simulink subsystem "AGTF30"  (R2021b)
settings: Solver=VariableStepAuto  StartTime=0.0  StopTime=10.0  RelTol=1e-3
undefined symbols (not defined in the file): MWS
libraries: Lib_Solve_IterNRSolverJC_TMATS x1
settings Model: Creator=prbalm  LastModifiedBy=prbalm

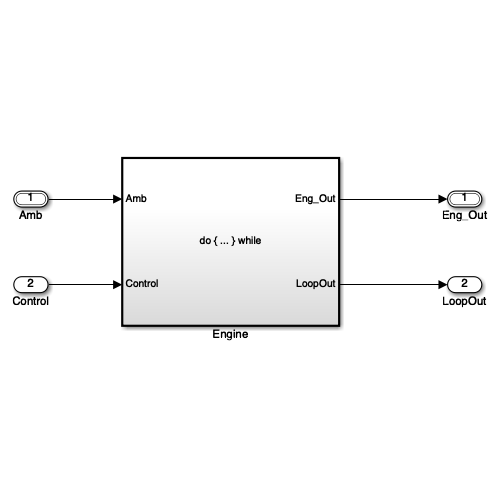
[thumbnail: Simulink's stored preview of the top-level diagram]
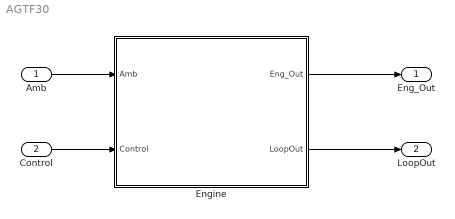
== system AGTF30 ==
  Amb : Inport
  Control : Inport  Port=2
  Engine : Subsystem
  Eng_Out : Outport  OutDataTypeStr=Bus: Eng_Bus
  LoopOut : Outport  Port=2
  wires:
  Engine/1(Eng_Out) -> Eng_Out/1
  Amb/1 -> Engine/1(Amb)
  Control/1 -> Engine/2(Control)
  Engine/2(LoopOut) -> LoopOut/1

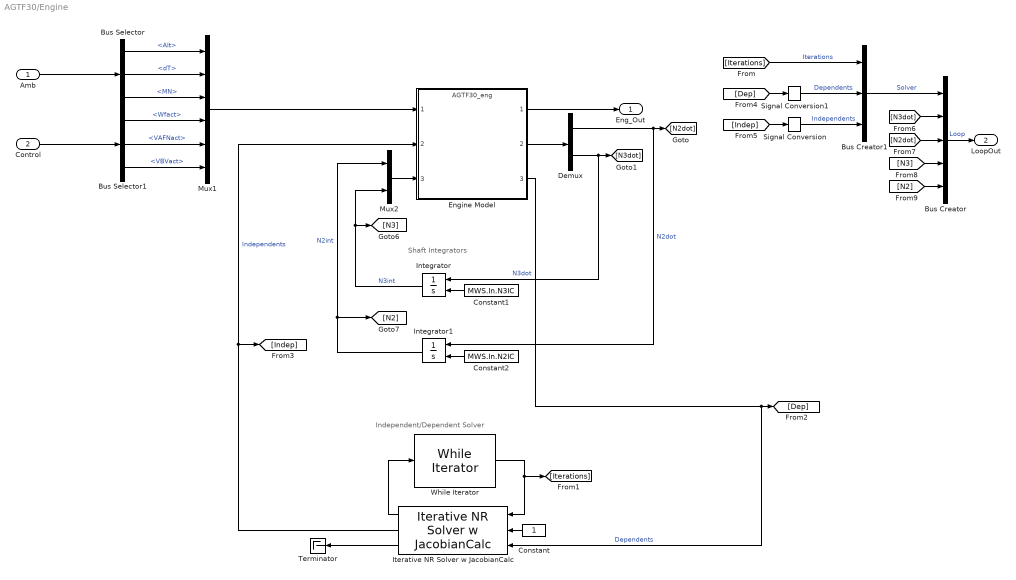
== system AGTF30/Engine ==
  note: Independent/Dependent Solver
  note: Shaft Integrators
  Amb : Inport
  Control : Inport  Port=2
  Bus Creator : BusCreator  Inputs=5
  Bus Creator1 : BusCreator  Inputs=3
  Bus Selector : BusSelector  OutputSignals=Alt,dT,MN
  Bus Selector1 : BusSelector  OutputSignals=Wfact,VAFNact,VBVact
  Constant : Constant
  Constant1 : Constant  Value=MWS.In.N3IC
  Constant2 : Constant  Value=MWS.In.N2IC
  Demux : Demux  Outputs=2
  Engine Model : ModelReference  ModelNameDialog=AGTF30_eng.mdl  SimulationMode=Normal  ModelReferenceVersion=1.306
  Integrator : Integrator  InitialConditionSource=external
  Integrator1 : Integrator  InitialConditionSource=external
  Iterative NR Solver w JacobianCalc : Lib_Solve_IterNRSolverJC_TMATS/Iterative NR Solver w JacobianCalc  SJac_Per_M=MWS.In.JPerDyn  SNR_IC_M=MWS.In.ICcom  SNR_DX_M=MWS.In.dX  SNR_Mx_M=100000  SNR_Mn_M=0.0001  SJacobianAttempts_M=MWS.In.NRADyn  Cond_Limits_M=MWS.In.Lim
  Mux1 : Mux  Inputs=6
  Mux2 : Mux  Inputs=2
  Signal Conversion : SignalConversion  OverrideOpt=off
  Signal Conversion1 : SignalConversion  OverrideOpt=off
  Terminator : Terminator
  While Iterator : WhileIterator  MaxIters=MWS.In.Max_IterDyn  WhileBlockType=do-while  ShowIterationPort=on
  Eng_Out : Outport
  LoopOut : Outport  Port=2
  wires:
  Constant2/1 -> Integrator1/2
  Constant1/1 -> Integrator/2
  Mux2/1 -> Engine Model/3
  Engine Model/2 -> Demux/1
  Mux1/1 -> Engine Model/1
  Engine Model/1 -> Eng_Out/1
  While Iterator/1 -> [Iterations], Iterative NR Solver w JacobianCalc/1
  Engine Model/3 -> [Dep], Iterative NR Solver w JacobianCalc/3  "Dependents"
  Iterative NR Solver w JacobianCalc/2 -> Engine Model/2, [Indep]  "Independents"
  Iterative NR Solver w JacobianCalc/3 -> Terminator/1
  Constant/1 -> Iterative NR Solver w JacobianCalc/2
  Iterative NR Solver w JacobianCalc/1 -> While Iterator/1
  [Indep] -> Signal Conversion/1
  Bus Creator1/1 -> Bus Creator/1  "Solver"
  Signal Conversion/1 -> Bus Creator1/3  "Independents"
  [Dep] -> Signal Conversion1/1
  [Iterations] -> Bus Creator1/1  "Iterations"
  Signal Conversion1/1 -> Bus Creator1/2  "Dependents"
  Demux/2 -> [N3dot], Integrator/1  "N3dot"
  Demux/1 -> [N2dot], Integrator1/1  "N2dot"
  Integrator1/1 -> Mux2/1, [N2]  "N2int"
  Integrator/1 -> Mux2/2, [N3]  "N3int"
  [N2] -> Bus Creator/5
  [N3] -> Bus Creator/4
  [N2dot] -> Bus Creator/3
  [N3dot] -> Bus Creator/2
  Bus Creator/1 -> LoopOut/1  "Loop"
  Bus Selector1/3 -> Mux1/6  "<VBVact>"
  Amb/1 -> Bus Selector/1
  Control/1 -> Bus Selector1/1
  Bus Selector/2 -> Mux1/2  "<dT>"
  Bus Selector/1 -> Mux1/1  "<Alt>"
  Bus Selector/3 -> Mux1/3  "<MN>"
  Bus Selector1/1 -> Mux1/4  "<Wfact>"
  Bus Selector1/2 -> Mux1/5  "<VAFNact>"
